simulink model "Simulacion_sistema_con_controlador_RL"  (R2021b)
settings: Solver=VariableStepAuto  StartTime=0.0  StopTime=20  FixedStep=0.01  RelTol=1e-3
model workspace (MATLAB code in the model file):
  | mCart = 1;
  | mPend = 1;
  | g = 9.81;
  | L = 0.5;
  | theta0 = 180;
  | Kd = 10;
values from neighbouring files (symbols this model uses):
  A = [0, 1, 0, 0;b4, 0, 0, b5;0, 0, 0, 1;b7, 0, 0, b8]    [Parametros_del_sistema_y_carga_del_agente_RL.m]
  B = [0;b6;0;b9]    [Parametros_del_sistema_y_carga_del_agente_RL.m]
  b4 = (b2*b3)/b10    (= 44.1287076335)    [Parametros_del_sistema_y_carga_del_agente_RL.m]
  b5 = [I2*a]/b10    [Parametros_del_sistema_y_carga_del_agente_RL.m]
  b6 = [-b*I2]/b10    [Parametros_del_sistema_y_carga_del_agente_RL.m]
  b7 = -[I2*c*b2]/b10    [Parametros_del_sistema_y_carga_del_agente_RL.m]
  b8 = -a*b1/b10    (= -2.72707287809)    [Parametros_del_sistema_y_carga_del_agente_RL.m]
  b9 = b*b1/b10    (= 16.0702508888)    [Parametros_del_sistema_y_carga_del_agente_RL.m]
  C = [1,0,0,0;0,0,1,0]    [Parametros_del_sistema_y_carga_del_agente_RL.m]
  Ke = [G*inv(X)]'    [Parametros_del_sistema_y_carga_del_agente_RL.m]
  Ts = 0.01    [Parametros_del_sistema_y_carga_del_agente_RL.m]
libraries: rllib x1
settings Model: Creator=The MathWorks, Inc.  LastModifiedBy=Antonio
settings SolverCC: AlgebraicLoopSolver=TrustRegion
settings DataIOCC: TimeSaveName=T  SignalLoggingName=LoggedSigs
settings DebuggingCC: SFMachineParentedDataDiag=warning  ArithmeticOperatorsInVariantConditions=warning
settings SFSimCC: CustomCodeUndefinedFunction=UseInterfaceOnly
settings RTWCC: DLArmComputeVersion=20.02.1

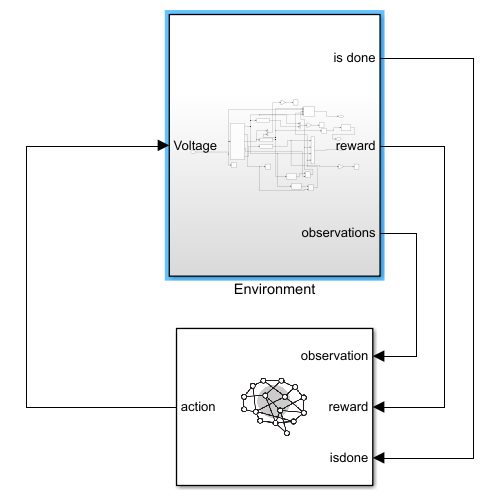
[thumbnail: Simulink's stored preview of the top-level diagram]
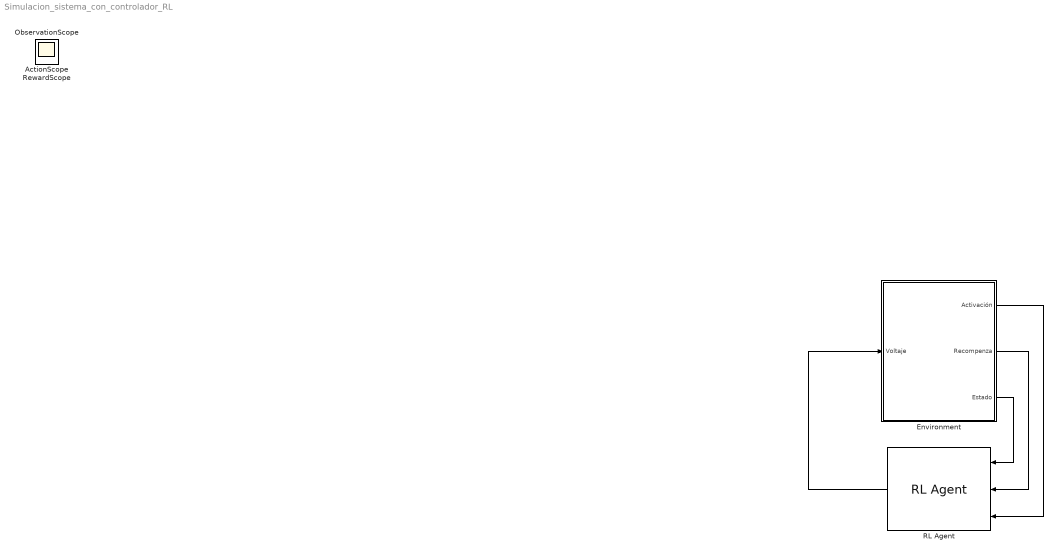
== system Simulacion_sistema_con_controlador_RL ==
  Environment : Subsystem
  RL Agent : rllib/RL Agent  Agent=agent  ExternalActionAsInput=off  ProvideCumRwd=off  TreatAsDirectFeedthrough=on
  ActionScope : Scope
  ObservationScope : Scope
  RewardScope : Scope
  wires:
  Environment/3(Estado) -> RL Agent/1
  Environment/2(Recompenza) -> RL Agent/2
  Environment/1(Activación) -> RL Agent/3
  RL Agent/1 -> Environment/1(Voltaje)

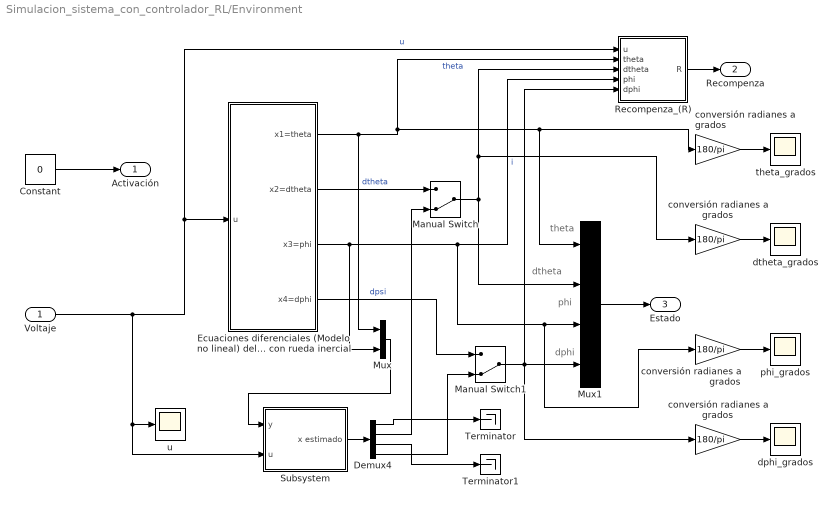
== system Simulacion_sistema_con_controlador_RL/Environment ==
  note: dphi
  note: phi
  note: dtheta
  note: theta
  Voltaje : Inport
  Constant : Constant  Value=0
  Demux4 : Demux
  Ecuaciones diferenciales (Modelo no lineal) del péndulo con rueda inercial : Subsystem
  Manual Switch : ManualSwitch  CurrentSetting=0
  Manual Switch1 : ManualSwitch  CurrentSetting=0
  Mux : Mux  Inputs=2
  Mux1 : Mux
  Recompenza_(R) : Subsystem
  Subsystem : Subsystem
  Terminator : Terminator
  Terminator1 : Terminator
  conversión radianes a grados : Gain  Gain=180/pi
  "conversión radianes a grados " : Gain  Gain=180/pi
  "conversión radianes a grados  " : Gain  Gain=180/pi
  "conversión radianes a grados   " : Gain  Gain=180/pi
  dphi_grados : Scope
  dtheta_grados : Scope
  phi_grados : Scope
  theta_grados : Scope
  u : Scope
  Activación : Outport  VectorParamsAs1DForOutWhenUnconnected=off
  Recompenza : Outport  Port=2  VectorParamsAs1DForOutWhenUnconnected=off
  Estado : Outport  Port=3  VectorParamsAs1DForOutWhenUnconnected=off
  wires:
  Mux1/1 -> Estado/1
  Ecuaciones diferenciales (Modelo no lineal) del péndulo con rueda inercial/3(x3=phi) -> Recompenza_(R)/4(phi), Mux1/3, "conversión radianes a grados "/1, Mux/2  "i"
  Voltaje/1 -> Recompenza_(R)/1(u), Ecuaciones diferenciales (Modelo no lineal) del péndulo con rueda inercial/1(u), u/1, Subsystem/2(u)  "u"
  conversión radianes a grados/1 -> theta_grados/1
  Recompenza_(R)/1(R) -> Recompenza/1
  Constant/1 -> Activación/1
  Ecuaciones diferenciales (Modelo no lineal) del péndulo con rueda inercial/1(x1=theta) -> Recompenza_(R)/2(theta), Mux1/1, conversión radianes a grados/1, Mux/1  "theta"
  "conversión radianes a grados  "/1 -> dtheta_grados/1
  "conversión radianes a grados "/1 -> phi_grados/1
  "conversión radianes a grados   "/1 -> dphi_grados/1
  Ecuaciones diferenciales (Modelo no lineal) del péndulo con rueda inercial/2(x2=dtheta) -> Manual Switch/1  "dtheta"
  Subsystem/1(x estimado) -> Demux4/1
  Demux4/2 -> Manual Switch/2
  Manual Switch/1 -> Recompenza_(R)/3(dtheta), "conversión radianes a grados  "/1, Mux1/2
  Ecuaciones diferenciales (Modelo no lineal) del péndulo con rueda inercial/4(x4=dphi) -> Manual Switch1/1  "dpsi"
  Demux4/4 -> Manual Switch1/2
  Manual Switch1/1 -> "conversión radianes a grados   "/1, Recompenza_(R)/5(dphi), Mux1/4
  Demux4/1 -> Terminator/1
  Demux4/3 -> Terminator1/1
  Mux/1 -> Subsystem/1(y)

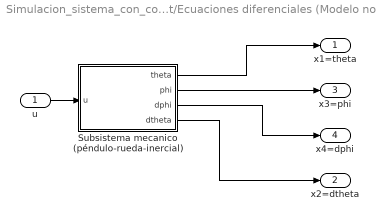
== system Simulacion_sistema_con_controlador_RL/Environment/Ecuaciones diferenciales (Modelo no lineal) del péndulo con rueda inercial ==
  u : Inport
  Subsistema mecanico (péndulo-rueda-inercial) : Subsystem
  x1=theta : Outport
  x2=dtheta : Outport  Port=2
  x3=phi : Outport  Port=3
  x4=dphi : Outport  Port=4
  wires:
  Subsistema mecanico (péndulo-rueda-inercial)/4(dtheta) -> x2=dtheta/1
  u/1 -> Subsistema mecanico (péndulo-rueda-inercial)/1(u)
  Subsistema mecanico (péndulo-rueda-inercial)/2(phi) -> x3=phi/1
  Subsistema mecanico (péndulo-rueda-inercial)/3(dphi) -> x4=dphi/1
  Subsistema mecanico (péndulo-rueda-inercial)/1(theta) -> x1=theta/1

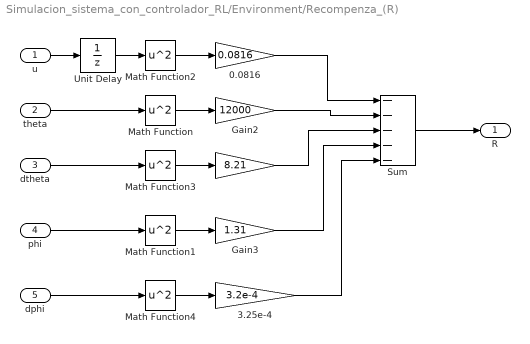
== system Simulacion_sistema_con_controlador_RL/Environment/Recompenza_(R) ==
  u : Inport
  theta : Inport  Port=2
  dtheta : Inport  Port=3
  phi : Inport  Port=4
  dphi : Inport  Port=5
  " " : Gain  Gain=8.21
  0.0816 : Gain  Gain=0.0816
  3.25e-4 : Gain  Gain=3.2e-4
  Gain2 : Gain  Gain=12000
  Gain3 : Gain  Gain=1.31
  Math Function{,1..4} (5 alike) : Math  Operator=square  SignedPower=on  SaturateOnIntegerOverflow=on
  Sum : Sum  Inputs=-----
  Unit Delay : UnitDelay  SampleTime=Ts  HasFrameUpgradeWarning=on
  R : Outport  VectorParamsAs1DForOutWhenUnconnected=off
  wires:
  theta/1 -> Math Function/1
  Gain2/1 -> Sum/2
  Math Function2/1 -> 0.0816/1
  Math Function1/1 -> Gain3/1
  u/1 -> Unit Delay/1
  phi/1 -> Math Function1/1
  Math Function/1 -> Gain2/1
  0.0816/1 -> Sum/1
  Unit Delay/1 -> Math Function2/1
  Sum/1 -> R/1
  Math Function3/1 -> " "/1
  dtheta/1 -> Math Function3/1
  dphi/1 -> Math Function4/1
  Math Function4/1 -> 3.25e-4/1
  3.25e-4/1 -> Sum/5
  " "/1 -> Sum/3
  Gain3/1 -> Sum/4

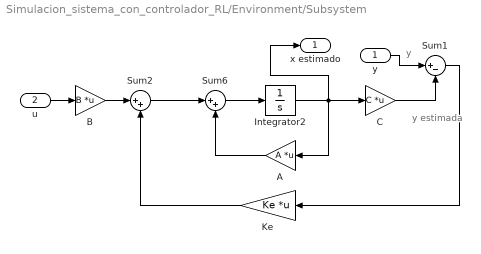
== system Simulacion_sistema_con_controlador_RL/Environment/Subsystem ==
  note: y
  note: y estimada
  y : Inport
  u : Inport  Port=2
  A : Gain  Gain=A  Multiplication=Matrix(K*u)
  B : Gain  Gain=B  Multiplication=Matrix(K*u)
  C : Gain  Gain=C  Multiplication=Matrix(K*u)
  Integrator2 : Integrator
  Ke : Gain  Gain=Ke  Multiplication=Matrix(K*u)
  Sum1 : Sum  Inputs=|+-
  Sum2 : Sum  Inputs=|++
  Sum6 : Sum  Inputs=|++
  x estimado : Outport
  wires:
  C/1 -> Sum1/2
  Integrator2/1 -> x estimado/1, A/1, C/1
  Sum2/1 -> Sum6/1
  Ke/1 -> Sum2/2
  B/1 -> Sum2/1
  Sum6/1 -> Integrator2/1
  Sum1/1 -> Ke/1
  A/1 -> Sum6/2
  y/1 -> Sum1/1
  u/1 -> B/1

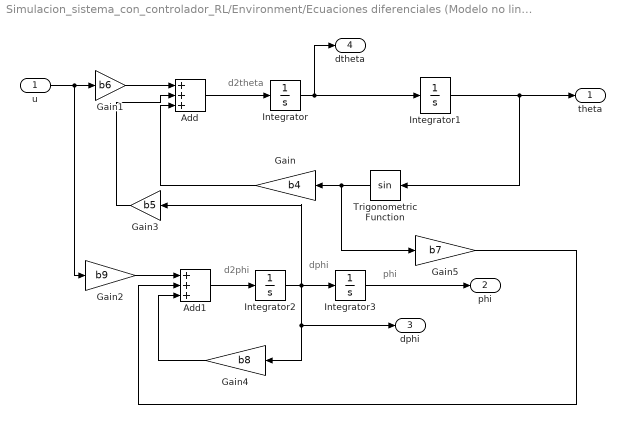
== system Simulacion_sistema_con_controlador_RL/Environment/Ecuaciones diferenciales (Modelo no lineal) del péndulo con rueda inercial/Subsistema mecanico (péndulo-rueda-inercial) ==
  note: d2theta
  note: phi
  note: dphi
  note: d2phi
  u : Inport
  Add : Sum  Inputs=+++
  Add1 : Sum  Inputs=+++
  Gain : Gain  Gain=b4
  Gain1 : Gain  Gain=b6
  Gain2 : Gain  Gain=b9
  Gain3 : Gain  Gain=b5
  Gain4 : Gain  Gain=b8
  Gain5 : Gain  Gain=b7
  Integrator : Integrator
  Integrator1 : Integrator  InitialCondition=-4*pi/180
  Integrator2 : Integrator
  Integrator3 : Integrator
  Trigonometric Function : Trigonometry
  theta : Outport
  phi : Outport  Port=2
  dphi : Outport  Port=3
  dtheta : Outport  Port=4
  wires:
  Add/1 -> Integrator/1
  Gain2/1 -> Add1/1
  Gain1/1 -> Add/1
  Add1/1 -> Integrator2/1
  Integrator1/1 -> Trigonometric Function/1, theta/1
  Integrator2/1 -> Gain3/1, dphi/1, Gain4/1, Integrator3/1
  u/1 -> Gain2/1, Gain1/1
  Trigonometric Function/1 -> Gain/1, Gain5/1
  Integrator3/1 -> phi/1
  Integrator/1 -> dtheta/1, Integrator1/1
  Gain/1 -> Add/3
  Gain3/1 -> Add/2
  Gain4/1 -> Add1/3
  Gain5/1 -> Add1/2
